simulink model "DOF4_model_v3"  (R2023a)
settings: Solver=FixedStepAuto  StartTime=0.0  StopTime=10.0  FixedStep=5e-3  RelTol=1e-3
values from neighbouring files (symbols this model uses):
  z_r_type = 1    [DOF_4_parameters.m]
undefined symbols (not defined in the file or in its folder): chassis, constants, suspension
libraries: simulink x1
settings Model: Creator=Cassio de Freitas  LastModifiedBy=Cassio de Freitas
settings DataIOCC: ReturnWorkspaceOutputsName=simout

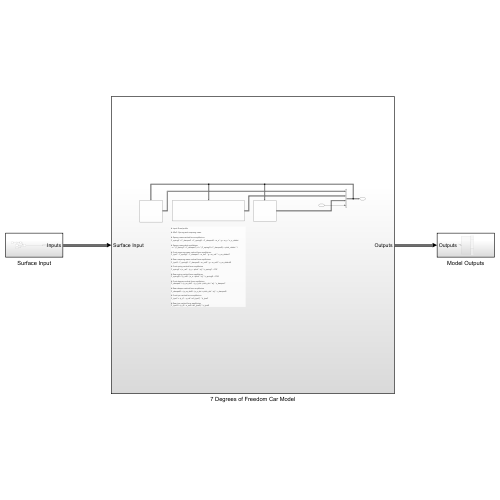
[thumbnail: Simulink's stored preview of the top-level diagram]
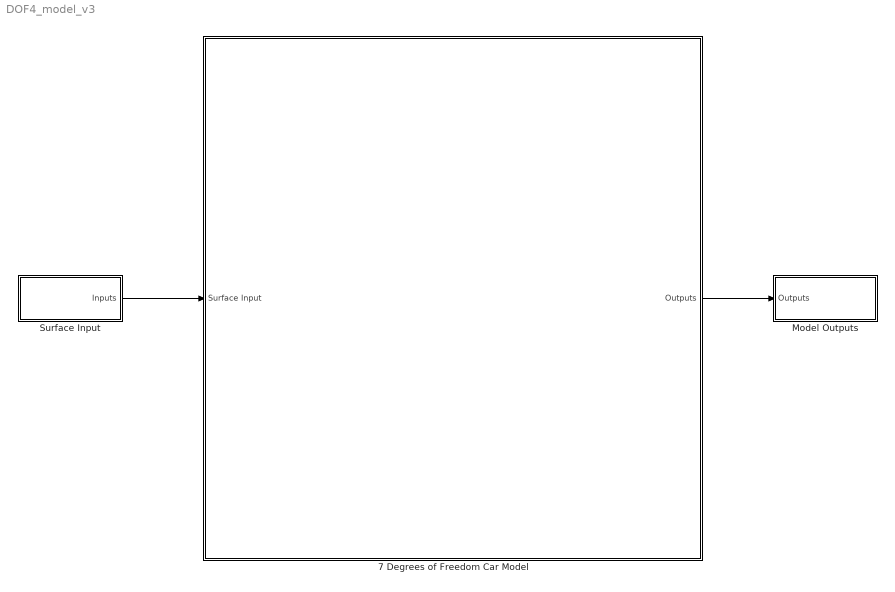
== system DOF4_model_v3 ==
  7 Degrees of Freedom Car Model : Subsystem
  Model Outputs : Subsystem
  Surface Input : Subsystem
  wires:
  7 Degrees of Freedom Car Model/1(Outputs) -> Model Outputs/1(Outputs)
  Surface Input/1(Inputs) -> 7 Degrees of Freedom Car Model/1(Surface Input)

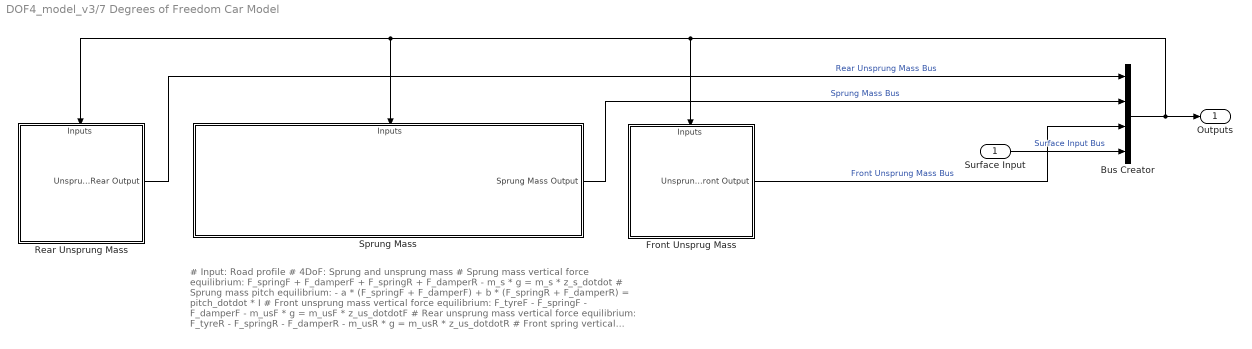
== system DOF4_model_v3/7 Degrees of Freedom Car Model ==
  note: # Input: Road profile
      |
      | # 4DoF: Sprung and unsprung mass
      |
      | # Sprung mass vertical force equilibrium:
      | F_springF + F_damperF + F_springR + F_damperR - m_s * g = m_s * z_s_dotdot
      |
      | # Sprung mass pitch equilibrium:
      | - a * (F_springF + F_damperF) + b * (F_springR + F_damperR) = pitch_dotdot * I
      |
      | # Front unsprung mass vertical force equilibrium:
      | F_tyreF - F_springF - F_damperF - m_usF * g = m_usF * z_us_dotdotF
      |
      | # Rear unsprung mass vertical force equilibrium:
      | F_tyreR - F_springR - F_damperR - m_usR * g = m_usR * z_us_dotdotR
      |
      | # Front spring vertical force equilibrium
      | F_springF = (z_usF - (z_s - pitch * a)) * k_springF + F0F
      |
      | # Rear spring vertical force equilibrium
      | F_springR = (z_usR - (z_s + pitch * b)) * k_springR + F0R
      |
      | # Front damper vertical force equilibrium
      | F_damperF = (z_us_dotF - (z_s_dot - pitch_dot * a)) * c_damperF
      |
      | # Rear damper vertical force equilibrium
      | F_damperR = (z_us_dotR - (z_s_dot + pitch_dot * a)) * c_damperR
      |
      | # Front tyre vertical force equilibrium
      | F_tyreF = (z_rF - z_usF +z0_tyreF) * k_tyreF
      |
      | # Rear tyre vertical force equilibrium
      | F_tyreR = (z_rR - z_usR +z0_tyreR) * k_tyreR
  Surface Input : Inport
  Bus Creator : BusCreator  Inputs=4
  Front Unsprug Mass : Subsystem
      settings: PortSchema="{\"entries\":[{\"content\":{\"sides\":[{\"content\":{},\"type\":\"ConnectorPlacement.EquallySpacedRectSide\",\"uuid\":\"ca30240c-8ef1-46c7-89f3-8e50ced18502\"},{\"content\":{\"connectorIds\":[\"Out1\"],\"side\":\"RIGHT\"},\"type\":\"ConnectorPlacement.EquallySpacedRectSide\",\"uuid\":\"c07c8638-1df4-45b7-a4a8-af2a14da671f\"},{\"content\":{\"connectorIds\":[\"In1\"],\"side\":\"TOP\"},\"type\":\"ConnectorPlacement.EquallySpacedRectSide\",\"uuid\":\"eabc6117-aa62-4f5e-810e-ab9c70bf779a\"}]},\"type\":\"ConnectorPlacement.EquallySpacedConnector\",\"uuid\":\"d3560202-2442-4eac-8aeb-f346a931fc21\"}],\"packageUris\":[\"http://schema.mathworks.com/mf0/Connector/R2020b\"],\"version\":\"1.0\"}"
  Rear Unsprung Mass : Subsystem
      settings: PortSchema="{\"entries\":[{\"content\":{\"sides\":[{\"content\":{},\"type\":\"ConnectorPlacement.EquallySpacedRectSide\",\"uuid\":\"ca30240c-8ef1-46c7-89f3-8e50ced18502\"},{\"content\":{\"connectorIds\":[\"Out1\"],\"side\":\"RIGHT\"},\"type\":\"ConnectorPlacement.EquallySpacedRectSide\",\"uuid\":\"c07c8638-1df4-45b7-a4a8-af2a14da671f\"},{\"content\":{\"connectorIds\":[\"In1\"],\"side\":\"TOP\"},\"type\":\"ConnectorPlacement.EquallySpacedRectSide\",\"uuid\":\"eabc6117-aa62-4f5e-810e-ab9c70bf779a\"}]},\"type\":\"ConnectorPlacement.EquallySpacedConnector\",\"uuid\":\"d3560202-2442-4eac-8aeb-f346a931fc21\"}],\"packageUris\":[\"http://schema.mathworks.com/mf0/Connector/R2020b\"],\"version\":\"1.0\"}"
  Sprung Mass : Subsystem
      settings: PortSchema="{\"entries\":[{\"content\":{\"sides\":[{\"content\":{},\"type\":\"ConnectorPlacement.EquallySpacedRectSide\",\"uuid\":\"63b5c35c-1345-4ade-85d7-a7aac4cc3700\"},{\"content\":{\"connectorIds\":[\"Out1\"],\"side\":\"RIGHT\"},\"type\":\"ConnectorPlacement.EquallySpacedRectSide\",\"uuid\":\"42c6bf5f-ecea-40ec-868a-6613098306c6\"},{\"content\":{\"connectorIds\":[\"In1\"],\"side\":\"TOP\"},\"type\":\"ConnectorPlacement.EquallySpacedRectSide\",\"uuid\":\"4661345b-8a90-4c28-8ce6-d1521a801330\"}]},\"type\":\"ConnectorPlacement.EquallySpacedConnector\",\"uuid\":\"31a4e6e8-77fc-45d3-842e-fbcb04573c93\"}],\"packageUris\":[\"http://schema.mathworks.com/mf0/Connector/R2020b\"],\"version\":\"1.0\"}"
  Outputs : Outport
  wires:
  Rear Unsprung Mass/1(Unsprung Mass Rear Output) -> Bus Creator/1  "Rear Unsprung Mass Bus"
  Sprung Mass/1(Sprung Mass Output) -> Bus Creator/2  "Sprung Mass Bus"
  Front Unsprug Mass/1(Unsprung Mass Front Output) -> Bus Creator/3  "Front Unsprung Mass Bus"
  Bus Creator/1 -> Front Unsprug Mass/1(Inputs), Rear Unsprung Mass/1(Inputs), Sprung Mass/1(Inputs), Outputs/1
  Surface Input/1 -> Bus Creator/4  "Surface Input Bus"

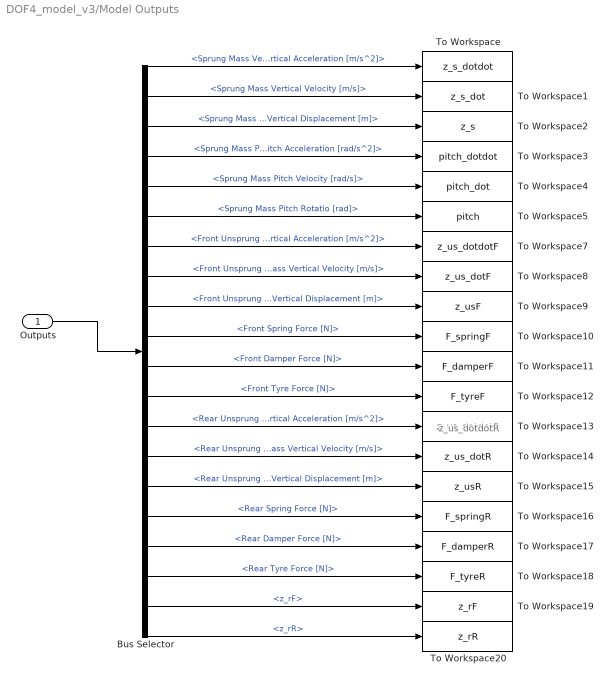
== system DOF4_model_v3/Model Outputs ==
  note: z_us_dotdotR
  Outputs : Inport
  Bus Selector : BusSelector  OutputSignals=Sprung Mass Bus.Sprung Mass Vertical Acceleration [m/s^2],Sprung Mass Bus.Sprung Mass Vertical Velocity [m/s],Sprung Mass Bus.Sprung Mass Vertical Displacement [m],Sprung Mass Bus.Sprung Mass Pitch Acceleration [rad/s^2],Sprung Mass Bus.Sprung Mass Pitch Velocity [rad/s],Sprung Mass Bus.Sprung Mass Pitch Rotatio [rad],Front Unsprung Mass Bus.Front Unsprung Mass Vertical Acceleration [m/s^2],Front Unsprung Mass Bus.Front Unsprung Mass Vertical Velocity [m/s],Front Unsprung Mass Bus.Front Unsprung Mass Vertical Displacement [m],Front Unsprung Mass Bus.Front Spring Force [N],Front Unsprung Mass Bus.Front Damper Force [N],Front Unsprung Mass Bus.Front Tyre Force [N],Rear Unsprung Mass Bus.Rear Unsprung Mass Vertical Acceleration [m/s^2],Rear Unsprung Mass Bus.Rear Unsprung Mass Vertical Velocity [m/s],Rear Unsprung Mass Bus.Rear Unsprung Mass Vertical Displacement [m],Rear Unsprung Mass Bus.Rear Spring Force [N],Rear Unsprung Mass Bus.Rear Damper Force [N],Rear Unsprung Mass Bus.Rear Tyre Force [N],Surface Input Bus.z_rF,Surface Input Bus.z_rR
  To Workspace : ToWorkspace  VariableName=z_s_dotdot  SaveFormat=Timeseries  SampleTime=-1
  To Workspace1 : ToWorkspace  VariableName=z_s_dot  SaveFormat=Timeseries  SampleTime=-1
  To Workspace10 : ToWorkspace  VariableName=F_springF  SaveFormat=Timeseries  SampleTime=-1
  To Workspace11 : ToWorkspace  VariableName=F_damperF  SaveFormat=Timeseries  SampleTime=-1
  To Workspace12 : ToWorkspace  VariableName=F_tyreF  SaveFormat=Timeseries  SampleTime=-1
  To Workspace13 : ToWorkspace  VariableName=z_us_dotdotR  SaveFormat=Timeseries  SampleTime=-1
  To Workspace14 : ToWorkspace  VariableName=z_us_dotR  SaveFormat=Timeseries  SampleTime=-1
  To Workspace15 : ToWorkspace  VariableName=z_usR  SaveFormat=Timeseries  SampleTime=-1
  To Workspace16 : ToWorkspace  VariableName=F_springR  SaveFormat=Timeseries  SampleTime=-1
  To Workspace17 : ToWorkspace  VariableName=F_damperR  SaveFormat=Timeseries  SampleTime=-1
  To Workspace18 : ToWorkspace  VariableName=F_tyreR  SaveFormat=Timeseries  SampleTime=-1
  To Workspace19 : ToWorkspace  VariableName=z_rF  SaveFormat=Timeseries  SampleTime=-1
  To Workspace2 : ToWorkspace  VariableName=z_s  SaveFormat=Timeseries  SampleTime=-1
  To Workspace20 : ToWorkspace  VariableName=z_rR  SaveFormat=Timeseries  SampleTime=-1
  To Workspace3 : ToWorkspace  VariableName=pitch_dotdot  SaveFormat=Timeseries  SampleTime=-1
  To Workspace4 : ToWorkspace  VariableName=pitch_dot  SaveFormat=Timeseries  SampleTime=-1
  To Workspace5 : ToWorkspace  VariableName=pitch  SaveFormat=Timeseries  SampleTime=-1
  To Workspace7 : ToWorkspace  VariableName=z_us_dotdotF  SaveFormat=Timeseries  SampleTime=-1
  To Workspace8 : ToWorkspace  VariableName=z_us_dotF  SaveFormat=Timeseries  SampleTime=-1
  To Workspace9 : ToWorkspace  VariableName=z_usF  SaveFormat=Timeseries  SampleTime=-1
  wires:
  Outputs/1 -> Bus Selector/1
  Bus Selector/1 -> To Workspace/1  "<Sprung Mass Vertical Acceleration [m/s^2]>"
  Bus Selector/2 -> To Workspace1/1  "<Sprung Mass Vertical Velocity [m/s]>"
  Bus Selector/3 -> To Workspace2/1  "<Sprung Mass Vertical Displacement [m]>"
  Bus Selector/4 -> To Workspace3/1  "<Sprung Mass Pitch Acceleration [rad/s^2]>"
  Bus Selector/5 -> To Workspace4/1  "<Sprung Mass Pitch Velocity [rad/s]>"
  Bus Selector/6 -> To Workspace5/1  "<Sprung Mass Pitch Rotatio [rad]>"
  Bus Selector/7 -> To Workspace7/1  "<Front Unsprung Mass Vertical Acceleration [m/s^2]>"
  Bus Selector/8 -> To Workspace8/1  "<Front Unsprung Mass Vertical Velocity [m/s]>"
  Bus Selector/9 -> To Workspace9/1  "<Front Unsprung Mass Vertical Displacement [m]>"
  Bus Selector/10 -> To Workspace10/1  "<Front Spring Force [N]>"
  Bus Selector/11 -> To Workspace11/1  "<Front Damper Force [N]>"
  Bus Selector/12 -> To Workspace12/1  "<Front Tyre Force [N]>"
  Bus Selector/13 -> To Workspace13/1  "<Rear Unsprung Mass Vertical Acceleration [m/s^2]>"
  Bus Selector/14 -> To Workspace14/1  "<Rear Unsprung Mass Vertical Velocity [m/s]>"
  Bus Selector/15 -> To Workspace15/1  "<Rear Unsprung Mass Vertical Displacement [m]>"
  Bus Selector/16 -> To Workspace16/1  "<Rear Spring Force [N]>"
  Bus Selector/17 -> To Workspace17/1  "<Rear Damper Force [N]>"
  Bus Selector/18 -> To Workspace18/1  "<Rear Tyre Force [N]>"
  Bus Selector/19 -> To Workspace19/1  "<z_rF>"
  Bus Selector/20 -> To Workspace20/1  "<z_rR>"

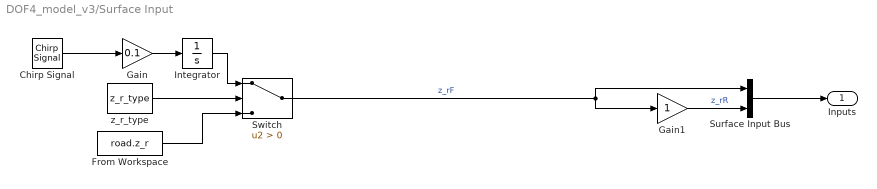
== system DOF4_model_v3/Surface Input ==
  Chirp Signal : simulink/Sources/Chirp Signal  f1=0.1  T=100  f2=50
  From Workspace : FromWorkspace  VariableName=road.z_r
  Gain : Gain  Gain=0.1
  Gain1 : Gain
  Integrator : Integrator
  Surface Input Bus : BusCreator  Inputs=2
  Switch : Switch  Criteria=u2 > Threshold  SaturateOnIntegerOverflow=off  InputSameDT=off
  z_r_type : Constant  Value=z_r_type
  Inputs : Outport
  wires:
  Switch/1 -> Gain1/1, Surface Input Bus/1  "z_rF"
  Integrator/1 -> Switch/1
  Gain/1 -> Integrator/1
  Chirp Signal/1 -> Gain/1
  z_r_type/1 -> Switch/2
  From Workspace/1 -> Switch/3
  Surface Input Bus/1 -> Inputs/1
  Gain1/1 -> Surface Input Bus/2  "z_rR"

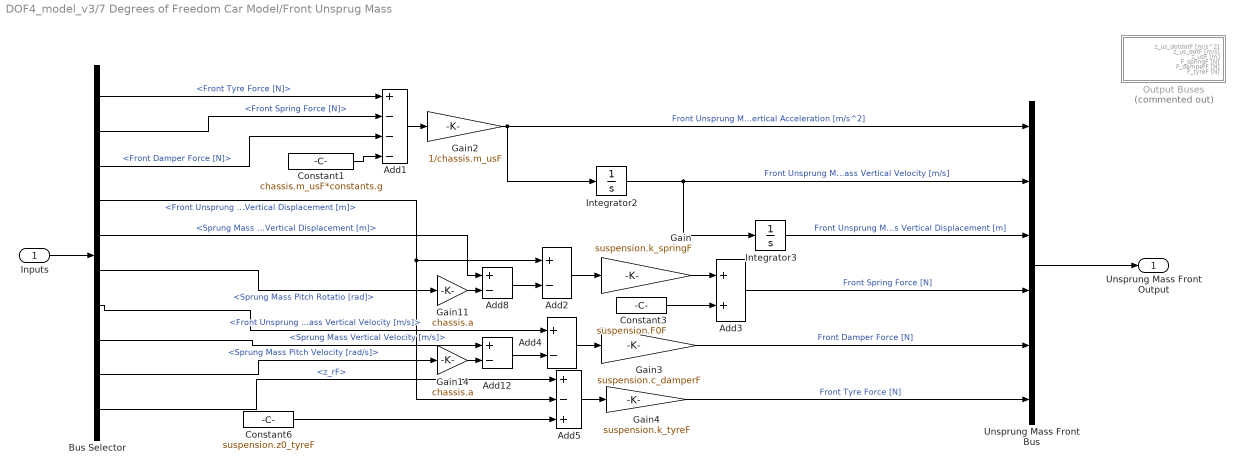
== system DOF4_model_v3/7 Degrees of Freedom Car Model/Front Unsprug Mass ==
  Inputs : Inport
  Add1 : Sum  Inputs=+---
  Add{2,4,8,12} (4 alike) : Sum  Inputs=+-
  Add3 : Sum
  Add5 : Sum  Inputs=+-+
  Bus Selector : BusSelector  OutputSignals=Front Unsprung Mass Bus.Front Tyre Force [N],Front Unsprung Mass Bus.Front Spring Force [N],Front Unsprung Mass Bus.Front Damper Force [N],Front Unsprung Mass Bus.Front Unsprung Mass Vertical Displacement [m],Sprung Mass Bus.Sprung Mass Vertical Displacement [m],Sprung Mass Bus.Sprung Mass Pitch Rotatio [rad],Front Unsprung Mass Bus.Front Unsprung Mass Vertical Velocity [m/s],Sprung Mass Bus.Sprung Mass Vertical Velocity [m/s],Sprung Mass Bus.Sprung Mass Pitch Velocity [rad/s],Surface Input Bus.z_rF
  Constant1 : Constant  Value=chassis.m_usF*constants.g
  Constant3 : Constant  Value=suspension.F0F
  Constant6 : Constant  Value=suspension.z0_tyreF
  Gain : Gain  Gain=suspension.k_springF
  Gain11 : Gain  Gain=chassis.a
  Gain14 : Gain  Gain=chassis.a
  Gain2 : Gain  Gain=1/chassis.m_usF
  Gain3 : Gain  Gain=suspension.c_damperF
  Gain4 : Gain  Gain=suspension.k_tyreF
  Integrator2 : Integrator
  Integrator3 : Integrator
  Output Buses : Subsystem  Commented=on
  Unsprung Mass Front Bus : BusCreator  Inputs=6
  Unsprung Mass Front Output : Outport
  wires:
  Integrator3/1 -> Unsprung Mass Front Bus/3  "Front Unsprung Mass Vertical Displacement [m]"
  Add1/1 -> Gain2/1
  Integrator2/1 -> Unsprung Mass Front Bus/2, Integrator3/1  "Front Unsprung Mass Vertical Velocity [m/s]"
  Gain2/1 -> Integrator2/1, Unsprung Mass Front Bus/1  "Front Unsprung Mass Vertical Acceleration [m/s^2]"
  Gain11/1 -> Add8/2
  Bus Selector/5 -> Add8/1  "<Sprung Mass Vertical Displacement [m]>"
  Add8/1 -> Add2/2
  Add3/1 -> Unsprung Mass Front Bus/4  "Front Spring Force [N]"
  Gain/1 -> Add3/1
  Add4/1 -> Gain3/1
  Constant3/1 -> Add3/2
  Bus Selector/4 -> Add5/2, Add2/1  "<Front Unsprung Mass Vertical Displacement [m]>"
  Gain3/1 -> Unsprung Mass Front Bus/5  "Front Damper Force [N]"
  Gain14/1 -> Add12/2
  Add2/1 -> Gain/1
  Add12/1 -> Add4/2
  Add5/1 -> Gain4/1
  Constant6/1 -> Add5/3
  Gain4/1 -> Unsprung Mass Front Bus/6  "Front Tyre Force [N]"
  Bus Selector/3 -> Add1/3  "<Front Damper Force [N]>"
  Bus Selector/1 -> Add1/1  "<Front Tyre Force [N]>"
  Constant1/1 -> Add1/4
  Bus Selector/7 -> Add4/1  "<Front Unsprung Mass Vertical Velocity [m/s]>"
  Bus Selector/9 -> Gain14/1  "<Sprung Mass Pitch Velocity [rad/s]>"
  Unsprung Mass Front Bus/1 -> Unsprung Mass Front Output/1
  Inputs/1 -> Bus Selector/1
  Bus Selector/2 -> Add1/2  "<Front Spring Force [N]>"
  Bus Selector/6 -> Gain11/1  "<Sprung Mass Pitch Rotatio [rad]>"
  Bus Selector/8 -> Add12/1  "<Sprung Mass Vertical Velocity [m/s]>"
  Bus Selector/10 -> Add5/1  "<z_rF>"

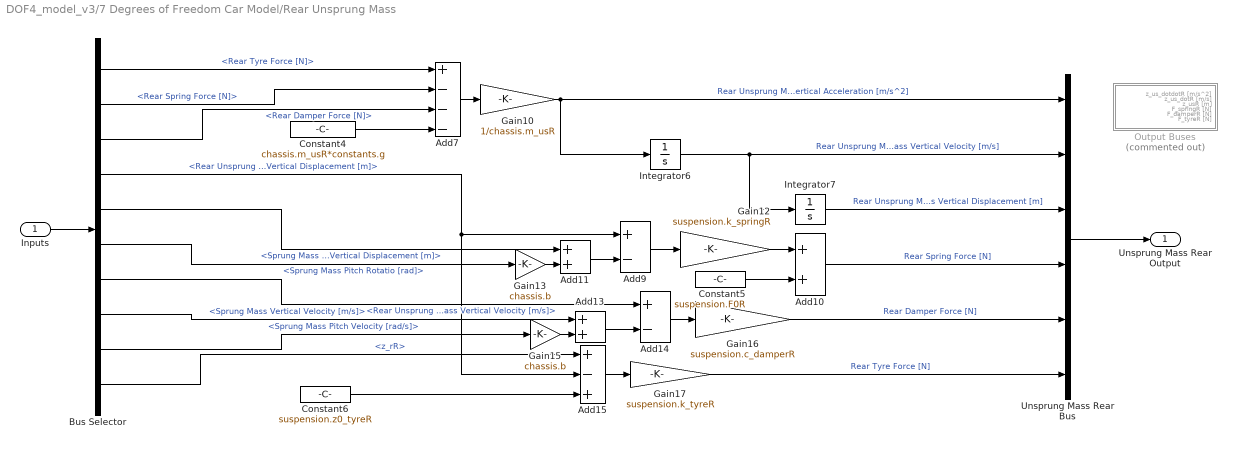
== system DOF4_model_v3/7 Degrees of Freedom Car Model/Rear Unsprung Mass ==
  Inputs : Inport
  Add10 : Sum
  Add11 : Sum
  Add13 : Sum
  Add14 : Sum  Inputs=+-
  Add15 : Sum  Inputs=+-+
  Add7 : Sum  Inputs=+---
  Add9 : Sum  Inputs=+-
  Bus Selector : BusSelector  OutputSignals=Rear Unsprung Mass Bus.Rear Tyre Force [N],Rear Unsprung Mass Bus.Rear Spring Force [N],Rear Unsprung Mass Bus.Rear Damper Force [N],Rear Unsprung Mass Bus.Rear Unsprung Mass Vertical Displacement [m],Sprung Mass Bus.Sprung Mass Vertical Displacement [m],Sprung Mass Bus.Sprung Mass Pitch Rotatio [rad],Rear Unsprung Mass Bus.Rear Unsprung Mass Vertical Velocity [m/s],Sprung Mass Bus.Sprung Mass Vertical Velocity [m/s],Sprung Mass Bus.Sprung Mass Pitch Velocity [rad/s],Surface Input Bus.z_rR
  Constant4 : Constant  Value=chassis.m_usR*constants.g
  Constant5 : Constant  Value=suspension.F0R
  Constant6 : Constant  Value=suspension.z0_tyreR
  Gain10 : Gain  Gain=1/chassis.m_usR
  Gain12 : Gain  Gain=suspension.k_springR
  Gain13 : Gain  Gain=chassis.b
  Gain15 : Gain  Gain=chassis.b
  Gain16 : Gain  Gain=suspension.c_damperR
  Gain17 : Gain  Gain=suspension.k_tyreR
  Integrator6 : Integrator
  Integrator7 : Integrator
  Output Buses : Subsystem  Commented=on
  Unsprung Mass Rear Bus : BusCreator  Inputs=6
  Unsprung Mass Rear Output : Outport
  wires:
  Integrator7/1 -> Unsprung Mass Rear Bus/3  "Rear Unsprung Mass Vertical Displacement [m]"
  Add7/1 -> Gain10/1
  Gain10/1 -> Integrator6/1, Unsprung Mass Rear Bus/1  "Rear Unsprung Mass Vertical Acceleration [m/s^2]"
  Integrator6/1 -> Unsprung Mass Rear Bus/2, Integrator7/1  "Rear Unsprung Mass Vertical Velocity [m/s]"
  Add11/1 -> Add9/2
  Add9/1 -> Gain12/1
  Gain16/1 -> Unsprung Mass Rear Bus/5  "Rear Damper Force [N]"
  Add13/1 -> Add14/2
  Gain13/1 -> Add11/2
  Gain12/1 -> Add10/1
  Add14/1 -> Gain16/1
  Add10/1 -> Unsprung Mass Rear Bus/4  "Rear Spring Force [N]"
  Gain15/1 -> Add13/2
  Constant5/1 -> Add10/2
  Gain17/1 -> Unsprung Mass Rear Bus/6  "Rear Tyre Force [N]"
  Add15/1 -> Gain17/1
  Bus Selector/1 -> Add7/1  "<Rear Tyre Force [N]>"
  Bus Selector/3 -> Add7/3  "<Rear Damper Force [N]>"
  Constant4/1 -> Add7/4
  Bus Selector/4 -> Add9/1, Add15/2  "<Rear Unsprung Mass Vertical Displacement [m]>"
  Bus Selector/5 -> Add11/1  "<Sprung Mass Vertical Displacement [m]>"
  Bus Selector/6 -> Gain13/1  "<Sprung Mass Pitch Rotatio [rad]>"
  Bus Selector/7 -> Add14/1  "<Rear Unsprung Mass Vertical Velocity [m/s]>"
  Bus Selector/8 -> Add13/1  "<Sprung Mass Vertical Velocity [m/s]>"
  Bus Selector/9 -> Gain15/1  "<Sprung Mass Pitch Velocity [rad/s]>"
  Bus Selector/10 -> Add15/1  "<z_rR>"
  Constant6/1 -> Add15/3
  Unsprung Mass Rear Bus/1 -> Unsprung Mass Rear Output/1
  Inputs/1 -> Bus Selector/1
  Bus Selector/2 -> Add7/2  "<Rear Spring Force [N]>"

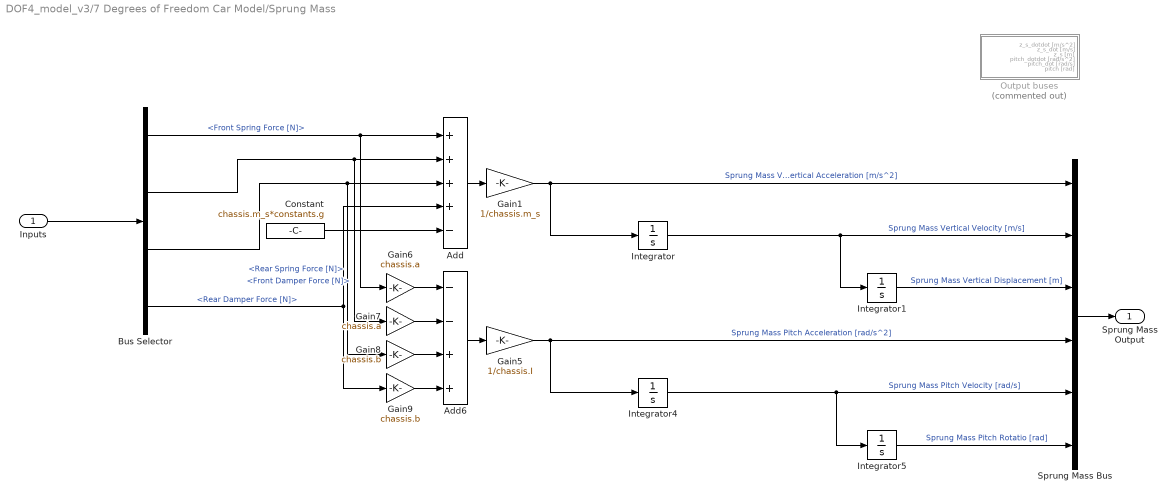
== system DOF4_model_v3/7 Degrees of Freedom Car Model/Sprung Mass ==
  Inputs : Inport
  Add : Sum  Inputs=++++-
  Add6 : Sum  Inputs=--++
  Bus Selector : BusSelector  OutputSignals=Front Unsprung Mass Bus.Front Spring Force [N],Front Unsprung Mass Bus.Front Damper Force [N],Rear Unsprung Mass Bus.Rear Spring Force [N],Rear Unsprung Mass Bus.Rear Damper Force [N]
  Constant : Constant  Value=chassis.m_s*constants.g
  Gain1 : Gain  Gain=1/chassis.m_s
  Gain5 : Gain  Gain=1/chassis.I
  Gain6 : Gain  Gain=chassis.a
  Gain7 : Gain  Gain=chassis.a
  Gain8 : Gain  Gain=chassis.b
  Gain9 : Gain  Gain=chassis.b
  Integrator{,1,4..5} (4 alike) : Integrator
  Output buses : Subsystem  Commented=on
  Sprung Mass Bus : BusCreator  Inputs=6
  Sprung Mass Output : Outport
  wires:
  Integrator4/1 -> Sprung Mass Bus/5, Integrator5/1  "Sprung Mass Pitch Velocity [rad/s]"
  Gain5/1 -> Integrator4/1, Sprung Mass Bus/4  "Sprung Mass Pitch Acceleration [rad/s^2]"
  Gain9/1 -> Add6/4
  Gain1/1 -> Integrator/1, Sprung Mass Bus/1  "Sprung Mass Vertical Acceleration [m/s^2]"
  Integrator1/1 -> Sprung Mass Bus/3  "Sprung Mass Vertical Displacement [m]"
  Add/1 -> Gain1/1
  Gain8/1 -> Add6/3
  Add6/1 -> Gain5/1
  Gain7/1 -> Add6/2
  Gain6/1 -> Add6/1
  Integrator5/1 -> Sprung Mass Bus/6  "Sprung Mass Pitch Rotatio [rad]"
  Integrator/1 -> Integrator1/1, Sprung Mass Bus/2  "Sprung Mass Vertical Velocity [m/s]"
  Bus Selector/1 -> Gain6/1, Add/1  "<Front Spring Force [N]>"
  Bus Selector/2 -> Gain7/1, Add/2  "<Front Damper Force [N]>"
  Bus Selector/3 -> Gain8/1, Add/3  "<Rear Spring Force [N]>"
  Bus Selector/4 -> Add/4, Gain9/1  "<Rear Damper Force [N]>"
  Constant/1 -> Add/5
  Sprung Mass Bus/1 -> Sprung Mass Output/1
  Inputs/1 -> Bus Selector/1

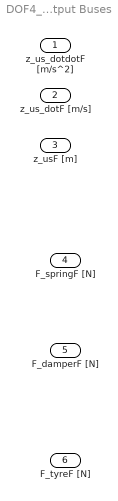
== system DOF4_model_v3/7 Degrees of Freedom Car Model/Front Unsprug Mass/Output Buses ==
  z_us_dotdotF [m/s^2] : Outport
  z_us_dotF [m/s] : Outport  Port=2
  z_usF [m] : Outport  Port=3
  F_springF [N] : Outport  Port=4
  F_damperF [N] : Outport  Port=5
  F_tyreF [N] : Outport  Port=6

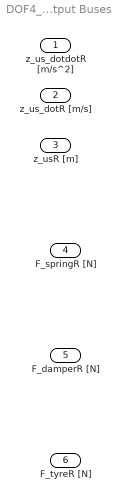
== system DOF4_model_v3/7 Degrees of Freedom Car Model/Rear Unsprung Mass/Output Buses ==
  z_us_dotdotR [m/s^2] : Outport
  z_us_dotR [m/s] : Outport  Port=2
  z_usR [m] : Outport  Port=3
  F_springR [N] : Outport  Port=4
  F_damperR [N] : Outport  Port=5
  F_tyreR [N] : Outport  Port=6

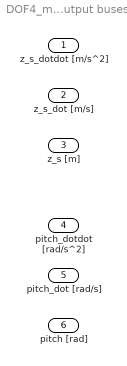
== system DOF4_model_v3/7 Degrees of Freedom Car Model/Sprung Mass/Output buses ==
  z_s_dotdot [m/s^2] : Outport
  z_s_dot [m/s] : Outport  Port=2
  z_s [m] : Outport  Port=3
  pitch_dotdot [rad/s^2] : Outport  Port=4
  pitch_dot [rad/s] : Outport  Port=5
  pitch [rad] : Outport  Port=6
